simulink model "EPT"  (R2019b)
settings: Solver=FixedStepDiscrete  StartTime=0.0  StopTime=5  FixedStep=0.005  RelTol=1e-3  EnableMultiTasking=on
PreLoadFcn:
  | try, model_open; catch, disp('Error occurred while executing model pre-load callback: model_open.m'); disp('Please assure that the MATLAB working directory is set to the model directory before opening.'); end
InitFcn:
  | try, model_open; catch, end
undefined symbols (not defined in the file or in its folder): Bridge, GCM, H, ln, raptor_get_param_eval, raptor_get_safe_string, raptor_xcp_function
libraries: Raptor_lib x2810, simulink x374, hdlsllib x19
(part 6 of 45)

== system EPT/I//O/Input/ADC_CoolingSystem  ==
  raptor_analog_in1 : Raptor_lib/Input & Output/raptor_analog_in  resourceValues=INPUT2|INPUT3|INPUT4|INPUT5|INPUT6|INPUT7|INPUT8|INPUT9|INPUT10|INPUT11|INPUT12|INPUT13|INPUT14|INPUT15|INPUT16|INPUT17|INPUT18|INPUT19|INPUT20|INPUT21|INPUT22|INPUT23|INPUT24|INPUT25|INPUT26|INPUT27|INPUT28|INPUT29|INPUT30|INPUT31|INPUT32|(None)  resource=INPUT19  pullUDValues=2.15k PU  pullUD=2.15k PU  rangeValues=0 - 5 V  range=0 - 5 V  filterrateValues=[]  filterrate='RAPTOR MASK DEFAULT'  resolutionValues=[]  resolution=[]
      settings: SourceProductName=Raptor
  raptor_analog_in2 : Raptor_lib/Input & Output/raptor_analog_in  resourceValues=INPUT2|INPUT3|INPUT4|INPUT5|INPUT6|INPUT7|INPUT8|INPUT9|INPUT10|INPUT11|INPUT12|INPUT13|INPUT14|INPUT15|INPUT16|INPUT17|INPUT18|INPUT19|INPUT20|INPUT21|INPUT22|INPUT23|INPUT24|INPUT25|INPUT26|INPUT27|INPUT28|INPUT29|INPUT30|INPUT31|INPUT32|(None)  resource=INPUT3  pullUDValues=2.15k PU  pullUD=2.15k PU  rangeValues=0 - 5 V  range=0 - 5 V  filterrateValues=[]  filterrate='RAPTOR MASK DEFAULT'  resolutionValues=[]  resolution=[]
      settings: SourceProductName=Raptor
  raptor_data_def6 : Raptor_lib/Data Storage/raptor_data_def  dataName='A105_Cooling_Oil_Temp_in'  initValue=0  dataType=uint16  storage=Volatile (RAM)  calVisible=on  calType=Measurement  calDispType=Number  calEnum={'False', 'True'}  calGain=1.0  calOffset=0  calMin=-inf  calMax=inf  calFormat='-1'  calUnit=''  calHelp=''  calAccess=1  calFunction=raptor_xcp_function(gcb)  calDispHeaders=off  calColHeaders={'Col1' 'Col2' 'Col3'}  calRowHeaders={'Row1' 'Row2' 'Row3'}
      settings: SourceProductName=Raptor
  raptor_data_def9 : Raptor_lib/Data Storage/raptor_data_def  dataName='A17_Cooling_Water_Temp_in'  initValue=0  dataType=uint16  storage=Volatile (RAM)  calVisible=on  calType=Measurement  calDispType=Number  calEnum={'False', 'True'}  calGain=1.0  calOffset=0  calMin=-inf  calMax=inf  calFormat='-1'  calUnit=''  calHelp=''  calAccess=1  calFunction=raptor_xcp_function(gcb)  calDispHeaders=off  calColHeaders={'Col1' 'Col2' 'Col3'}  calRowHeaders={'Row1' 'Row2' 'Row3'}
      settings: SourceProductName=Raptor
  raptor_data_write2 : Raptor_lib/Data Storage/raptor_data_write  dataName='A17_Cooling_Water_Temp_in'  dataShape=Scalar  idxSource=Input Port  idxRow=1  idxCol=1
      settings: SourceProductName=Raptor
  raptor_data_write4 : Raptor_lib/Data Storage/raptor_data_write  dataName='A105_Cooling_Oil_Temp_in'  dataShape=Scalar  idxSource=Input Port  idxRow=1  idxCol=1
      settings: SourceProductName=Raptor
  wires:
  raptor_analog_in2/1 -> raptor_data_write2/1
  raptor_analog_in1/1 -> raptor_data_write4/1

== system EPT/I//O/Input/ADC_PlugOn ==
  raptor_analog_in : Raptor_lib/Input & Output/raptor_analog_in  resourceValues=INPUT2|INPUT3|INPUT4|INPUT5|INPUT6|INPUT7|INPUT8|INPUT9|INPUT10|INPUT11|INPUT12|INPUT13|INPUT14|INPUT15|INPUT16|INPUT17|INPUT18|INPUT19|INPUT20|INPUT21|INPUT22|INPUT23|INPUT24|INPUT25|INPUT26|INPUT27|INPUT28|INPUT29|INPUT30|INPUT31|INPUT32|(None)  resource=INPUT5  pullUDValues=681k PU  pullUD=681k PU  rangeValues=0 - 5 V  range=0 - 5 V  filterrateValues=[]  filterrate='RAPTOR MASK DEFAULT'  resolutionValues=[]  resolution=[]
      settings: SourceProductName=Raptor
  raptor_analog_in1 : Raptor_lib/Input & Output/raptor_analog_in  resourceValues=INPUT2|INPUT3|INPUT4|INPUT5|INPUT6|INPUT7|INPUT8|INPUT9|INPUT10|INPUT11|INPUT12|INPUT13|INPUT14|INPUT15|INPUT16|INPUT17|INPUT18|INPUT19|INPUT20|INPUT21|INPUT22|INPUT23|INPUT24|INPUT25|INPUT26|INPUT27|INPUT28|INPUT29|INPUT30|INPUT31|INPUT32|(None)  resource=INPUT6  pullUDValues=681k PU  pullUD=681k PU  rangeValues=0 - 5 V  range=0 - 5 V  filterrateValues=[]  filterrate='RAPTOR MASK DEFAULT'  resolutionValues=[]  resolution=[]
      settings: SourceProductName=Raptor
  raptor_measurement : Raptor_lib/Data Storage/raptor_measurement  paramName='A19_PON_SW_G2'  nameSource=Parameter  calDispType=Number  calEnum={'False', 'True'}  calGain=1.0  calOffset=0.0  calMax=inf  calMin=-inf  calFormat='-1'  calUnit=''  calHelp=''  calAccess=1  calFunction=raptor_xcp_function(gcb)  calVisible=on
      settings: SourceProductName=Raptor
  raptor_measurement1 : Raptor_lib/Data Storage/raptor_measurement  paramName='A37_PON_SW_G1'  nameSource=Parameter  calDispType=Number  calEnum={'False', 'True'}  calGain=1.0  calOffset=0.0  calMax=inf  calMin=-inf  calFormat='-1'  calUnit=''  calHelp=''  calAccess=1  calFunction=raptor_xcp_function(gcb)  calVisible=on
      settings: SourceProductName=Raptor
  wires:
  raptor_analog_in/1 -> raptor_measurement/1
  raptor_analog_in1/1 -> raptor_measurement1/1

== system EPT/I//O/Input/ADC_Reserved ==
  raptor_analog_in2 : Raptor_lib/Input & Output/raptor_analog_in  resourceValues=INPUT2|INPUT3|INPUT4|INPUT5|INPUT6|INPUT7|INPUT8|INPUT9|INPUT10|INPUT11|INPUT12|INPUT13|INPUT14|INPUT15|INPUT16|INPUT17|INPUT18|INPUT19|INPUT20|INPUT21|INPUT22|INPUT23|INPUT24|INPUT25|INPUT26|INPUT27|INPUT28|INPUT29|INPUT30|INPUT31|INPUT32|(None)  resource=INPUT8  pullUDValues=4.64k PU  pullUD=4.64k PU  rangeValues=0 - 5 V  range=0 - 5 V  filterrateValues=[]  filterrate='RAPTOR MASK DEFAULT'  resolutionValues=[]  resolution=[]
      settings: SourceProductName=Raptor
  raptor_analog_in3 : Raptor_lib/Input & Output/raptor_analog_in  resourceValues=INPUT2|INPUT3|INPUT4|INPUT5|INPUT6|INPUT7|INPUT8|INPUT9|INPUT10|INPUT11|INPUT12|INPUT13|INPUT14|INPUT15|INPUT16|INPUT17|INPUT18|INPUT19|INPUT20|INPUT21|INPUT22|INPUT23|INPUT24|INPUT25|INPUT26|INPUT27|INPUT28|INPUT29|INPUT30|INPUT31|INPUT32|(None)  resource=INPUT21  pullUDValues=2.15k PU  pullUD=2.15k PU  rangeValues=0 - 5 V  range=0 - 5 V  filterrateValues=[]  filterrate='RAPTOR MASK DEFAULT'  resolutionValues=[]  resolution=[]
      settings: SourceProductName=Raptor
  raptor_analog_in4 : Raptor_lib/Input & Output/raptor_analog_in  resourceValues=INPUT2|INPUT3|INPUT4|INPUT5|INPUT6|INPUT7|INPUT8|INPUT9|INPUT10|INPUT11|INPUT12|INPUT13|INPUT14|INPUT15|INPUT16|INPUT17|INPUT18|INPUT19|INPUT20|INPUT21|INPUT22|INPUT23|INPUT24|INPUT25|INPUT26|INPUT27|INPUT28|INPUT29|INPUT30|INPUT31|INPUT32|(None)  resource=INPUT29  pullUDValues=215k PD  pullUD=215k PD  rangeValues=0 - 5 V  range=0 - 5 V  filterrateValues=[]  filterrate='RAPTOR MASK DEFAULT'  resolutionValues=[]  resolution=[]
      settings: SourceProductName=Raptor
  raptor_measurement2 : Raptor_lib/Data Storage/raptor_measurement  paramName='A40_Position1'  nameSource=Parameter  calDispType=Number  calEnum={'False', 'True'}  calGain=1.0  calOffset=0.0  calMax=inf  calMin=-inf  calFormat='-1'  calUnit=''  calHelp=''  calAccess=1  calFunction=raptor_xcp_function(gcb)  calVisible=on
      settings: SourceProductName=Raptor
  raptor_measurement3 : Raptor_lib/Data Storage/raptor_measurement  paramName='K13_Position2'  nameSource=Parameter  calDispType=Number  calEnum={'False', 'True'}  calGain=1.0  calOffset=0.0  calMax=inf  calMin=-inf  calFormat='-1'  calUnit=''  calHelp=''  calAccess=1  calFunction=raptor_xcp_function(gcb)  calVisible=on
      settings: SourceProductName=Raptor
  raptor_measurement4 : Raptor_lib/Data Storage/raptor_measurement  paramName='K65_Mode_1'  nameSource=Parameter  calDispType=Number  calEnum={'False', 'True'}  calGain=1.0  calOffset=0.0  calMax=inf  calMin=-inf  calFormat='-1'  calUnit=''  calHelp=''  calAccess=1  calFunction=raptor_xcp_function(gcb)  calVisible=on
      settings: SourceProductName=Raptor
  wires:
  raptor_analog_in2/1 -> raptor_measurement2/1
  raptor_analog_in3/1 -> raptor_measurement3/1
  raptor_analog_in4/1 -> raptor_measurement4/1

== system EPT/I//O/Input/ADC_TemperatureBatteryPack ==
  raptor_analog_in : Raptor_lib/Input & Output/raptor_analog_in  resourceValues=INPUT2|INPUT3|INPUT4|INPUT5|INPUT6|INPUT7|INPUT8|INPUT9|INPUT10|INPUT11|INPUT12|INPUT13|INPUT14|INPUT15|INPUT16|INPUT17|INPUT18|INPUT19|INPUT20|INPUT21|INPUT22|INPUT23|INPUT24|INPUT25|INPUT26|INPUT27|INPUT28|INPUT29|INPUT30|INPUT31|INPUT32|(None)  resource=INPUT22  pullUDValues=2.15k PU  pullUD=2.15k PU  rangeValues=0 - 5 V  range=0 - 5 V  filterrateValues=[]  filterrate='RAPTOR MASK DEFAULT'  resolutionValues=[]  resolution=[]
      settings: SourceProductName=Raptor
  raptor_analog_in1 : Raptor_lib/Input & Output/raptor_analog_in  resourceValues=INPUT2|INPUT3|INPUT4|INPUT5|INPUT6|INPUT7|INPUT8|INPUT9|INPUT10|INPUT11|INPUT12|INPUT13|INPUT14|INPUT15|INPUT16|INPUT17|INPUT18|INPUT19|INPUT20|INPUT21|INPUT22|INPUT23|INPUT24|INPUT25|INPUT26|INPUT27|INPUT28|INPUT29|INPUT30|INPUT31|INPUT32|(None)  resource=INPUT25  pullUDValues=2.15k PU  pullUD=2.15k PU  rangeValues=0 - 5 V  range=0 - 5 V  filterrateValues=[]  filterrate='RAPTOR MASK DEFAULT'  resolutionValues=[]  resolution=[]
      settings: SourceProductName=Raptor
  raptor_analog_in2 : Raptor_lib/Input & Output/raptor_analog_in  resourceValues=INPUT2|INPUT3|INPUT4|INPUT5|INPUT6|INPUT7|INPUT8|INPUT9|INPUT10|INPUT11|INPUT12|INPUT13|INPUT14|INPUT15|INPUT16|INPUT17|INPUT18|INPUT19|INPUT20|INPUT21|INPUT22|INPUT23|INPUT24|INPUT25|INPUT26|INPUT27|INPUT28|INPUT29|INPUT30|INPUT31|INPUT32|(None)  resource=INPUT27  pullUDValues=2.15k PU  pullUD=2.15k PU  rangeValues=0 - 5 V  range=0 - 5 V  filterrateValues=[]  filterrate='RAPTOR MASK DEFAULT'  resolutionValues=[]  resolution=[]
      settings: SourceProductName=Raptor
  raptor_analog_in3 : Raptor_lib/Input & Output/raptor_analog_in  resourceValues=INPUT2|INPUT3|INPUT4|INPUT5|INPUT6|INPUT7|INPUT8|INPUT9|INPUT10|INPUT11|INPUT12|INPUT13|INPUT14|INPUT15|INPUT16|INPUT17|INPUT18|INPUT19|INPUT20|INPUT21|INPUT22|INPUT23|INPUT24|INPUT25|INPUT26|INPUT27|INPUT28|INPUT29|INPUT30|INPUT31|INPUT32|(None)  resource=INPUT28  pullUDValues=2.15k PU  pullUD=2.15k PU  rangeValues=0 - 5 V  range=0 - 5 V  filterrateValues=[]  filterrate='RAPTOR MASK DEFAULT'  resolutionValues=[]  resolution=[]
      settings: SourceProductName=Raptor
  raptor_data_def : Raptor_lib/Data Storage/raptor_data_def  dataName='TBP_2'  initValue=0  dataType=uint16  storage=Volatile (RAM)  calVisible=on  calType=Measurement  calDispType=Number  calEnum={'False', 'True'}  calGain=1.0  calOffset=0  calMin=-inf  calMax=inf  calFormat='-1'  calUnit=''  calHelp=''  calAccess=1  calFunction=raptor_xcp_function(gcb)  calDispHeaders=off  calColHeaders={'Col1' 'Col2' 'Col3'}  calRowHeaders={'Row1' 'Row2' 'Row3'}
      settings: SourceProductName=Raptor
  raptor_data_def1 : Raptor_lib/Data Storage/raptor_data_def  dataName='TBP_1'  initValue=0  dataType=uint16  storage=Volatile (RAM)  calVisible=on  calType=Measurement  calDispType=Number  calEnum={'False', 'True'}  calGain=1.0  calOffset=0  calMin=-inf  calMax=inf  calFormat='-1'  calUnit=''  calHelp=''  calAccess=1  calFunction=raptor_xcp_function(gcb)  calDispHeaders=off  calColHeaders={'Col1' 'Col2' 'Col3'}  calRowHeaders={'Row1' 'Row2' 'Row3'}
      settings: SourceProductName=Raptor
  raptor_data_def2 : Raptor_lib/Data Storage/raptor_data_def  dataName='TBP_3'  initValue=0  dataType=uint16  storage=Volatile (RAM)  calVisible=on  calType=Measurement  calDispType=Number  calEnum={'False', 'True'}  calGain=1.0  calOffset=0  calMin=-inf  calMax=inf  calFormat='-1'  calUnit=''  calHelp=''  calAccess=1  calFunction=raptor_xcp_function(gcb)  calDispHeaders=off  calColHeaders={'Col1' 'Col2' 'Col3'}  calRowHeaders={'Row1' 'Row2' 'Row3'}
      settings: SourceProductName=Raptor
  raptor_data_def3 : Raptor_lib/Data Storage/raptor_data_def  dataName='TBP_4'  initValue=0  dataType=uint16  storage=Volatile (RAM)  calVisible=on  calType=Measurement  calDispType=Number  calEnum={'False', 'True'}  calGain=1.0  calOffset=0  calMin=-inf  calMax=inf  calFormat='-1'  calUnit=''  calHelp=''  calAccess=1  calFunction=raptor_xcp_function(gcb)  calDispHeaders=off  calColHeaders={'Col1' 'Col2' 'Col3'}  calRowHeaders={'Row1' 'Row2' 'Row3'}
      settings: SourceProductName=Raptor
  raptor_data_write1 : Raptor_lib/Data Storage/raptor_data_write  dataName='TBP_1'  dataShape=Scalar  idxSource=Input Port  idxRow=1  idxCol=1
      settings: SourceProductName=Raptor
  raptor_data_write2 : Raptor_lib/Data Storage/raptor_data_write  dataName='TBP_2'  dataShape=Scalar  idxSource=Input Port  idxRow=1  idxCol=1
      settings: SourceProductName=Raptor
  raptor_data_write3 : Raptor_lib/Data Storage/raptor_data_write  dataName='TBP_3'  dataShape=Scalar  idxSource=Input Port  idxRow=1  idxCol=1
      settings: SourceProductName=Raptor
  raptor_data_write4 : Raptor_lib/Data Storage/raptor_data_write  dataName='TBP_4'  dataShape=Scalar  idxSource=Input Port  idxRow=1  idxCol=1
      settings: SourceProductName=Raptor
  raptor_measurement : Raptor_lib/Data Storage/raptor_measurement  paramName='K30_TBP_1'  nameSource=Parameter  calDispType=Number  calEnum={'False', 'True'}  calGain=1.0  calOffset=0.0  calMax=inf  calMin=-inf  calFormat='-1'  calUnit=''  calHelp=''  calAccess=1  calFunction=raptor_xcp_function(gcb)  calVisible=on
      settings: SourceProductName=Raptor
  raptor_measurement1 : Raptor_lib/Data Storage/raptor_measurement  paramName='K42_TBP_2'  nameSource=Parameter  calDispType=Number  calEnum={'False', 'True'}  calGain=1.0  calOffset=0.0  calMax=inf  calMin=-inf  calFormat='-1'  calUnit=''  calHelp=''  calAccess=1  calFunction=raptor_xcp_function(gcb)  calVisible=on
      settings: SourceProductName=Raptor
  raptor_measurement2 : Raptor_lib/Data Storage/raptor_measurement  paramName='K51_TBP_3'  nameSource=Parameter  calDispType=Number  calEnum={'False', 'True'}  calGain=1.0  calOffset=0.0  calMax=inf  calMin=-inf  calFormat='-1'  calUnit=''  calHelp=''  calAccess=1  calFunction=raptor_xcp_function(gcb)  calVisible=on
      settings: SourceProductName=Raptor
  raptor_measurement3 : Raptor_lib/Data Storage/raptor_measurement  paramName='K58_TBP_4'  nameSource=Parameter  calDispType=Number  calEnum={'False', 'True'}  calGain=1.0  calOffset=0.0  calMax=inf  calMin=-inf  calFormat='-1'  calUnit=''  calHelp=''  calAccess=1  calFunction=raptor_xcp_function(gcb)  calVisible=on
      settings: SourceProductName=Raptor
  wires:
  raptor_analog_in/1 -> raptor_data_write1/1, raptor_measurement/1
  raptor_analog_in3/1 -> raptor_data_write4/1, raptor_measurement3/1
  raptor_analog_in2/1 -> raptor_measurement2/1, raptor_data_write3/1
  raptor_analog_in1/1 -> raptor_measurement1/1, raptor_data_write2/1

== system EPT/I//O/Input/Curtis_Reserved  ==
  raptor_analog_in : Raptor_lib/Input & Output/raptor_analog_in  resourceValues=INPUT2|INPUT3|INPUT4|INPUT5|INPUT6|INPUT7|INPUT8|INPUT9|INPUT10|INPUT11|INPUT12|INPUT13|INPUT14|INPUT15|INPUT16|INPUT17|INPUT18|INPUT19|INPUT20|INPUT21|INPUT22|INPUT23|INPUT24|INPUT25|INPUT26|INPUT27|INPUT28|INPUT29|INPUT30|INPUT31|INPUT32|(None)  resource=INPUT11  pullUDValues=681k PU  pullUD=681k PU  rangeValues=0 - 5 V  range=0 - 5 V  filterrateValues=[]  filterrate='RAPTOR MASK DEFAULT'  resolutionValues=[]  resolution=[]
      settings: SourceProductName=Raptor
  raptor_freq_in : Raptor_lib/Input & Output/raptor_freq_in  resourceValues=INPUT41|INPUT42|INPUT43|INPUT44|INPUT45|(None)  resource=INPUT42  hasDuty=on  pullUDValues=[]  pullUD=[]  interfaceValues=[]  interface=[]  hasEdgeCount='RAPTOR MASK DEFAULT'  filterValues=[]  filter=[]
      settings: SourceProductName=Raptor
  raptor_freq_in1 : Raptor_lib/Input & Output/raptor_freq_in  resourceValues=INPUT41|INPUT42|INPUT43|INPUT44|INPUT45|(None)  resource=INPUT45  hasDuty=on  pullUDValues=[]  pullUD=[]  interfaceValues=[]  interface=[]  hasEdgeCount='RAPTOR MASK DEFAULT'  filterValues=[]  filter=[]
      settings: SourceProductName=Raptor
  raptor_measurement : Raptor_lib/Data Storage/raptor_measurement  paramName='A55_MCU_Mode'  nameSource=Parameter  calDispType=Number  calEnum={'False', 'True'}  calGain=1.0  calOffset=0.0  calMax=inf  calMin=-inf  calFormat='-1'  calUnit=''  calHelp=''  calAccess=1  calFunction=raptor_xcp_function(gcb)  calVisible=on
      settings: SourceProductName=Raptor
  raptor_measurement1 : Raptor_lib/Data Storage/raptor_measurement  paramName='K18_Freq_MrpmA'  nameSource=Parameter  calDispType=Number  calEnum={'False', 'True'}  calGain=1.0  calOffset=0.0  calMax=inf  calMin=-inf  calFormat='-1'  calUnit=''  calHelp=''  calAccess=1  calFunction=raptor_xcp_function(gcb)  calVisible=on
      settings: SourceProductName=Raptor
  raptor_measurement2 : Raptor_lib/Data Storage/raptor_measurement  paramName='K52_Freq_MrpmB'  nameSource=Parameter  calDispType=Number  calEnum={'False', 'True'}  calGain=1.0  calOffset=0.0  calMax=inf  calMin=-inf  calFormat='-1'  calUnit=''  calHelp=''  calAccess=1  calFunction=raptor_xcp_function(gcb)  calVisible=on
      settings: SourceProductName=Raptor
  raptor_measurement3 : Raptor_lib/Data Storage/raptor_measurement  paramName='K18_Duty_MrpmA'  nameSource=Parameter  calDispType=Number  calEnum={'False', 'True'}  calGain=1.0  calOffset=0.0  calMax=inf  calMin=-inf  calFormat='-1'  calUnit=''  calHelp=''  calAccess=1  calFunction=raptor_xcp_function(gcb)  calVisible=on
      settings: SourceProductName=Raptor
  raptor_measurement5 : Raptor_lib/Data Storage/raptor_measurement  paramName='K52_Duty_MrpmB'  nameSource=Parameter  calDispType=Number  calEnum={'False', 'True'}  calGain=1.0  calOffset=0.0  calMax=inf  calMin=-inf  calFormat='-1'  calUnit=''  calHelp=''  calAccess=1  calFunction=raptor_xcp_function(gcb)  calVisible=on
      settings: SourceProductName=Raptor
  wires:
  raptor_analog_in/1 -> raptor_measurement/1
  raptor_freq_in/1 -> raptor_measurement1/1
  raptor_freq_in1/1 -> raptor_measurement2/1
  raptor_freq_in/2 -> raptor_measurement3/1
  raptor_freq_in1/2 -> raptor_measurement5/1

== system EPT/I//O/Output/BatteryPack_RelayControl  ==
  raptor_data_def16 : Raptor_lib/Data Storage/raptor_data_def  dataName='Flag_HV_Negative_Relay_On'  initValue=0  dataType=boolean  storage=Volatile (RAM)  calVisible=on  calType=Measurement  calDispType=Number  calEnum={'False', 'True'}  calGain=1.0  calOffset=0  calMin=-inf  calMax=inf  calFormat='-1'  calUnit=''  calHelp=''  calAccess=1  calFunction=raptor_xcp_function(gcb)  calDispHeaders=off  calColHeaders={'Col1' 'Col2' 'Col3'}  calRowHeaders={'Row1' 'Row2' 'Row3'}
      settings: SourceProductName=Raptor
  raptor_data_def17 : Raptor_lib/Data Storage/raptor_data_def  dataName='Flag_HV_Drive_Relay_On'  initValue=0  dataType=boolean  storage=Volatile (RAM)  calVisible=on  calType=Measurement  calDispType=Number  calEnum={'False', 'True'}  calGain=1.0  calOffset=0  calMin=-inf  calMax=inf  calFormat='-1'  calUnit=''  calHelp=''  calAccess=1  calFunction=raptor_xcp_function(gcb)  calDispHeaders=off  calColHeaders={'Col1' 'Col2' 'Col3'}  calRowHeaders={'Row1' 'Row2' 'Row3'}
      settings: SourceProductName=Raptor
  raptor_data_def18 : Raptor_lib/Data Storage/raptor_data_def  dataName='Flag_PreCharge_Relay_On'  initValue=0  dataType=boolean  storage=Volatile (RAM)  calVisible=on  calType=Measurement  calDispType=Number  calEnum={'False', 'True'}  calGain=1.0  calOffset=0  calMin=-inf  calMax=inf  calFormat='-1'  calUnit=''  calHelp=''  calAccess=1  calFunction=raptor_xcp_function(gcb)  calDispHeaders=off  calColHeaders={'Col1' 'Col2' 'Col3'}  calRowHeaders={'Row1' 'Row2' 'Row3'}
      settings: SourceProductName=Raptor
  raptor_data_def19 : Raptor_lib/Data Storage/raptor_data_def  dataName='Flag_Charger_Relay_On'  initValue=0  dataType=boolean  storage=Volatile (RAM)  calVisible=on  calType=Measurement  calDispType=Number  calEnum={'False', 'True'}  calGain=1.0  calOffset=0  calMin=-inf  calMax=inf  calFormat='-1'  calUnit=''  calHelp=''  calAccess=1  calFunction=raptor_xcp_function(gcb)  calDispHeaders=off  calColHeaders={'Col1' 'Col2' 'Col3'}  calRowHeaders={'Row1' 'Row2' 'Row3'}
      settings: SourceProductName=Raptor
  raptor_data_read1 : Raptor_lib/Data Storage/raptor_data_read  dataName='Flag_HV_Drive_Relay_On'  dataShape=Scalar  idxSource=Input  idxRow=1  idxCol=1
      settings: SourceProductName=Raptor
  raptor_data_read2 : Raptor_lib/Data Storage/raptor_data_read  dataName='Flag_PreCharge_Relay_On'  dataShape=Scalar  idxSource=Input  idxRow=1  idxCol=1
      settings: SourceProductName=Raptor
  raptor_data_read3 : Raptor_lib/Data Storage/raptor_data_read  dataName='Flag_Charger_Relay_On'  dataShape=Scalar  idxSource=Input  idxRow=1  idxCol=1
      settings: SourceProductName=Raptor
  raptor_data_read4 : Raptor_lib/Data Storage/raptor_data_read  dataName='Flag_HV_Negative_Relay_On'  dataShape=Scalar  idxSource=Input  idxRow=1  idxCol=1
      settings: SourceProductName=Raptor
  raptor_digital_out : Raptor_lib/Input & Output/raptor_digital_out  resourceValues=OUTPUT1|OUTPUT2|OUTPUT3|OUTPUT4|OUTPUT5|OUTPUT6|OUTPUT7|OUTPUT8|OUTPUT9|OUTPUT10|OUTPUT11|OUTPUT12|OUTPUT21|OUTPUT22|OUTPUT23|OUTPUT24|OUTPUT25|OUTPUT26|OUTPUT27|OUTPUT28|OUTPUT29|OUTPUT30|OUTPUT31|OUTPUT32|OUTPUT33|OUTPUT34|OUTPUT35|OUTPUT36|OUTPUT37|OUTPUT38|OUTPUT39|OUTPUT40|OUTPUT41|OUTPUT42|OUTPUT43|OUTPUT44|OUTPUT45|OUTPUT46|OUTPUT47|OUTPUT48|OUTPUT49|POWER_HOLD|(None)  resource=OUTPUT9  driverTypeValues=Low Side  driverType=Low Side
      settings: SourceProductName=Raptor
  raptor_digital_out1 : Raptor_lib/Input & Output/raptor_digital_out  resourceValues=OUTPUT1|OUTPUT2|OUTPUT3|OUTPUT4|OUTPUT5|OUTPUT6|OUTPUT7|OUTPUT8|OUTPUT9|OUTPUT10|OUTPUT11|OUTPUT12|OUTPUT21|OUTPUT22|OUTPUT23|OUTPUT24|OUTPUT25|OUTPUT26|OUTPUT27|OUTPUT28|OUTPUT29|OUTPUT30|OUTPUT31|OUTPUT32|OUTPUT33|OUTPUT34|OUTPUT35|OUTPUT36|OUTPUT37|OUTPUT38|OUTPUT39|OUTPUT40|OUTPUT41|OUTPUT42|OUTPUT43|OUTPUT44|OUTPUT45|OUTPUT46|OUTPUT47|OUTPUT48|OUTPUT49|POWER_HOLD|(None)  resource=OUTPUT12  driverTypeValues=Low Side  driverType=Low Side
      settings: SourceProductName=Raptor
  raptor_digital_out2 : Raptor_lib/Input & Output/raptor_digital_out  resourceValues=OUTPUT1|OUTPUT2|OUTPUT3|OUTPUT4|OUTPUT5|OUTPUT6|OUTPUT7|OUTPUT8|OUTPUT9|OUTPUT10|OUTPUT11|OUTPUT12|OUTPUT21|OUTPUT22|OUTPUT23|OUTPUT24|OUTPUT25|OUTPUT26|OUTPUT27|OUTPUT28|OUTPUT29|OUTPUT30|OUTPUT31|OUTPUT32|OUTPUT33|OUTPUT34|OUTPUT35|OUTPUT36|OUTPUT37|OUTPUT38|OUTPUT39|OUTPUT40|OUTPUT41|OUTPUT42|OUTPUT43|OUTPUT44|OUTPUT45|OUTPUT46|OUTPUT47|OUTPUT48|OUTPUT49|POWER_HOLD|(None)  resource=OUTPUT10  driverTypeValues=Low Side  driverType=Low Side
      settings: SourceProductName=Raptor
  raptor_digital_out3 : Raptor_lib/Input & Output/raptor_digital_out  resourceValues=OUTPUT1|OUTPUT2|OUTPUT3|OUTPUT4|OUTPUT5|OUTPUT6|OUTPUT7|OUTPUT8|OUTPUT9|OUTPUT10|OUTPUT11|OUTPUT12|OUTPUT21|OUTPUT22|OUTPUT23|OUTPUT24|OUTPUT25|OUTPUT26|OUTPUT27|OUTPUT28|OUTPUT29|OUTPUT30|OUTPUT31|OUTPUT32|OUTPUT33|OUTPUT34|OUTPUT35|OUTPUT36|OUTPUT37|OUTPUT38|OUTPUT39|OUTPUT40|OUTPUT41|OUTPUT42|OUTPUT43|OUTPUT44|OUTPUT45|OUTPUT46|OUTPUT47|OUTPUT48|OUTPUT49|POWER_HOLD|(None)  resource=OUTPUT21  driverTypeValues=Low Side  driverType=Low Side
      settings: SourceProductName=Raptor
  raptor_override1 : Raptor_lib/Data Storage/raptor_override  paramName='Cal_Relay_Drive'  nameSource=Parameter  measurement=None  calDispType=Number  calEnum={'False', 'True'}  calGain=1.0  calOffset=0.0  calMax=inf  calMin=-inf  calFormat='-1'  calUnit=''  calHelp=''  calAccess=1  calFunction=[raptor_xcp_function(gcb) '|' raptor_get_param_eval(gcb, 'paramName') '_Override']
      settings: SourceProductName=Raptor
  raptor_override2 : Raptor_lib/Data Storage/raptor_override  paramName='Cal_Relay_HV_Negative'  nameSource=Parameter  measurement=None  calDispType=Number  calEnum={'False', 'True'}  calGain=1.0  calOffset=0.0  calMax=inf  calMin=-inf  calFormat='-1'  calUnit=''  calHelp=''  calAccess=1  calFunction=[raptor_xcp_function(gcb) '|' raptor_get_param_eval(gcb, 'paramName') '_Override']
      settings: SourceProductName=Raptor
  raptor_override3 : Raptor_lib/Data Storage/raptor_override  paramName='Cal_Relay_PreChg'  nameSource=Parameter  measurement=None  calDispType=Number  calEnum={'False', 'True'}  calGain=1.0  calOffset=0.0  calMax=inf  calMin=-inf  calFormat='-1'  calUnit=''  calHelp=''  calAccess=1  calFunction=[raptor_xcp_function(gcb) '|' raptor_get_param_eval(gcb, 'paramName') '_Override']
      settings: SourceProductName=Raptor
  raptor_override4 : Raptor_lib/Data Storage/raptor_override  paramName='Cal_Relay_CHG'  nameSource=Parameter  measurement=None  calDispType=Number  calEnum={'False', 'True'}  calGain=1.0  calOffset=0.0  calMax=inf  calMin=-inf  calFormat='-1'  calUnit=''  calHelp=''  calAccess=1  calFunction=[raptor_xcp_function(gcb) '|' raptor_get_param_eval(gcb, 'paramName') '_Override']
      settings: SourceProductName=Raptor
  wires:
  raptor_data_read4/1 -> raptor_override2/1
  raptor_data_read2/1 -> raptor_override3/1
  raptor_override2/1 -> raptor_digital_out/1
  raptor_data_read1/1 -> raptor_override1/1
  raptor_override3/1 -> raptor_digital_out2/1
  raptor_override4/1 -> raptor_digital_out3/1
  raptor_data_read3/1 -> raptor_override4/1
  raptor_override1/1 -> raptor_digital_out1/1

== system EPT/I//O/Output/ChargerPlugInterface ==
  note: CHG Enable
  note: EOC Enable
  raptor_data_def13 : Raptor_lib/Data Storage/raptor_data_def  dataName='A24_EOC_Enable'  initValue=0  dataType=boolean  storage=Volatile (RAM)  calVisible=on  calType=Measurement  calDispType=Number  calEnum={'False', 'True'}  calGain=1.0  calOffset=0  calMin=-inf  calMax=inf  calFormat='-1'  calUnit=''  calHelp=''  calAccess=1  calFunction=raptor_xcp_function(gcb)  calDispHeaders=off  calColHeaders={'Col1' 'Col2' 'Col3'}  calRowHeaders={'Row1' 'Row2' 'Row3'}
      settings: SourceProductName=Raptor
  raptor_data_def14 : Raptor_lib/Data Storage/raptor_data_def  dataName='A10_CHG_Enable'  initValue=0  dataType=boolean  storage=Volatile (RAM)  calVisible=on  calType=Measurement  calDispType=Number  calEnum={'False', 'True'}  calGain=1.0  calOffset=0  calMin=-inf  calMax=inf  calFormat='-1'  calUnit=''  calHelp=''  calAccess=1  calFunction=raptor_xcp_function(gcb)  calDispHeaders=off  calColHeaders={'Col1' 'Col2' 'Col3'}  calRowHeaders={'Row1' 'Row2' 'Row3'}
      settings: SourceProductName=Raptor
  raptor_data_read1 : Raptor_lib/Data Storage/raptor_data_read  dataName='A24_EOC_Enable'  dataShape=Scalar  idxSource=Input  idxRow=1  idxCol=1
      settings: SourceProductName=Raptor
  raptor_data_read4 : Raptor_lib/Data Storage/raptor_data_read  dataName='A10_CHG_Enable'  dataShape=Scalar  idxSource=Input  idxRow=1  idxCol=1
      settings: SourceProductName=Raptor
  raptor_digital_out3 : Raptor_lib/Input & Output/raptor_digital_out  resourceValues=OUTPUT1|OUTPUT2|OUTPUT3|OUTPUT4|OUTPUT5|OUTPUT6|OUTPUT7|OUTPUT8|OUTPUT9|OUTPUT10|OUTPUT11|OUTPUT12|OUTPUT21|OUTPUT22|OUTPUT23|OUTPUT24|OUTPUT25|OUTPUT26|OUTPUT27|OUTPUT28|OUTPUT29|OUTPUT30|OUTPUT31|OUTPUT32|OUTPUT33|OUTPUT34|OUTPUT35|OUTPUT36|OUTPUT37|OUTPUT38|OUTPUT39|OUTPUT40|OUTPUT41|OUTPUT42|OUTPUT43|OUTPUT44|OUTPUT45|OUTPUT46|OUTPUT47|OUTPUT48|OUTPUT49|POWER_HOLD|(None)  resource=OUTPUT1  driverTypeValues=Low Side  driverType=Low Side
      settings: SourceProductName=Raptor
  raptor_digital_out4 : Raptor_lib/Input & Output/raptor_digital_out  resourceValues=OUTPUT1|OUTPUT2|OUTPUT3|OUTPUT4|OUTPUT5|OUTPUT6|OUTPUT7|OUTPUT8|OUTPUT9|OUTPUT10|OUTPUT11|OUTPUT12|OUTPUT21|OUTPUT22|OUTPUT23|OUTPUT24|OUTPUT25|OUTPUT26|OUTPUT27|OUTPUT28|OUTPUT29|OUTPUT30|OUTPUT31|OUTPUT32|OUTPUT33|OUTPUT34|OUTPUT35|OUTPUT36|OUTPUT37|OUTPUT38|OUTPUT39|OUTPUT40|OUTPUT41|OUTPUT42|OUTPUT43|OUTPUT44|OUTPUT45|OUTPUT46|OUTPUT47|OUTPUT48|OUTPUT49|POWER_HOLD|(None)  resource=OUTPUT3  driverTypeValues=Low Side  driverType=Low Side
      settings: SourceProductName=Raptor
  raptor_override : Raptor_lib/Data Storage/raptor_override  paramName='Cal_CHG_Enable'  nameSource=Parameter  measurement=None  calDispType=Number  calEnum={'False', 'True'}  calGain=1.0  calOffset=0.0  calMax=inf  calMin=-inf  calFormat='-1'  calUnit=''  calHelp=''  calAccess=1  calFunction=[raptor_xcp_function(gcb) '|' raptor_get_param_eval(gcb, 'paramName') '_Override']
      settings: SourceProductName=Raptor
  raptor_override1 : Raptor_lib/Data Storage/raptor_override  paramName='Cal_EOC_Enable'  nameSource=Parameter  measurement=None  calDispType=Number  calEnum={'False', 'True'}  calGain=1.0  calOffset=0.0  calMax=inf  calMin=-inf  calFormat='-1'  calUnit=''  calHelp=''  calAccess=1  calFunction=[raptor_xcp_function(gcb) '|' raptor_get_param_eval(gcb, 'paramName') '_Override']
      settings: SourceProductName=Raptor
  wires:
  raptor_data_read4/1 -> raptor_override/1
  raptor_data_read1/1 -> raptor_override1/1
  raptor_override/1 -> raptor_digital_out3/1
  raptor_override1/1 -> raptor_digital_out4/1

== system EPT/I//O/Output/Cooling System ==
  note: Motor Cooling
  note: OIL COOLER FAN
  note: WATER COOLER FAN
  note: MOTOR COOLER PW
  note: PACK COOLER PW
  note: Pack Cooling
  note: OIL COOLER FAN
  note: OIL PUMP
  note: WATER PUMP
  Data Type Conversion{,1..5} (6 alike) : DataTypeConversion
  Gain1 : Gain  Gain=100  OutDataTypeStr=uint32
  Gain2 : Gain  Gain=100  OutDataTypeStr=uint16
  Gain3 : Gain  Gain=100  OutDataTypeStr=uint32
  Gain4 : Gain  Gain=100  OutDataTypeStr=uint16
  Gain5 : Gain  Gain=100  OutDataTypeStr=uint32
  Gain6 : Gain  Gain=100  OutDataTypeStr=uint16
  raptor_adjustment1 : Raptor_lib/Data Storage/raptor_adjustment  paramName='K88_LSD_PWM_Freq'  nameSource=Parameter  initValue=1000  dataType=uint32  storage=Calibration  calDispType=Number  calEnum={'False', 'True'}  calGain=1.0  calOffset=0.0  calMax=inf  calMin=-inf  calFormat='-1'  calUnit=''  calHelp=''  calAccess=1  calFunction=raptor_xcp_function(gcb)  calDispHeaders=off  calColHeaders={'Col1' 'Col2' 'Col3'}  calRowHeaders={'Row1' 'Row2' 'Row3'}
      settings: SourceProductName=Raptor
  raptor_adjustment2 : Raptor_lib/Data Storage/raptor_adjustment  paramName='K88_LSD_PWM_EN'  nameSource=Parameter  initValue=1  dataType=boolean  storage=Calibration  calDispType=Number  calEnum={'False', 'True'}  calGain=1.0  calOffset=0.0  calMax=inf  calMin=-inf  calFormat='-1'  calUnit=''  calHelp=''  calAccess=1  calFunction=raptor_xcp_function(gcb)  calDispHeaders=off  calColHeaders={'Col1' 'Col2' 'Col3'}  calRowHeaders={'Row1' 'Row2' 'Row3'}
      settings: SourceProductName=Raptor
  raptor_adjustment3 : Raptor_lib/Data Storage/raptor_adjustment  paramName='A93_LSD_PWM_EN'  nameSource=Parameter  initValue=1  dataType=boolean  storage=Calibration  calDispType=Number  calEnum={'False', 'True'}  calGain=1.0  calOffset=0.0  calMax=inf  calMin=-inf  calFormat='-1'  calUnit=''  calHelp=''  calAccess=1  calFunction=raptor_xcp_function(gcb)  calDispHeaders=off  calColHeaders={'Col1' 'Col2' 'Col3'}  calRowHeaders={'Row1' 'Row2' 'Row3'}
      settings: SourceProductName=Raptor
  raptor_adjustment6 : Raptor_lib/Data Storage/raptor_adjustment  paramName='A23_LSD_PWM_Freq'  nameSource=Parameter  initValue=1000  dataType=uint32  storage=Calibration  calDispType=Number  calEnum={'False', 'True'}  calGain=1.0  calOffset=0.0  calMax=inf  calMin=-inf  calFormat='-1'  calUnit=''  calHelp=''  calAccess=1  calFunction=raptor_xcp_function(gcb)  calDispHeaders=off  calColHeaders={'Col1' 'Col2' 'Col3'}  calRowHeaders={'Row1' 'Row2' 'Row3'}
      settings: SourceProductName=Raptor
  raptor_adjustment7 : Raptor_lib/Data Storage/raptor_adjustment  paramName='A23_LSD_PWM_EN'  nameSource=Parameter  initValue=1  dataType=boolean  storage=Calibration  calDispType=Number  calEnum={'False', 'True'}  calGain=1.0  calOffset=0.0  calMax=inf  calMin=-inf  calFormat='-1'  calUnit=''  calHelp=''  calAccess=1  calFunction=raptor_xcp_function(gcb)  calDispHeaders=off  calColHeaders={'Col1' 'Col2' 'Col3'}  calRowHeaders={'Row1' 'Row2' 'Row3'}
      settings: SourceProductName=Raptor
  raptor_adjustment8 : Raptor_lib/Data Storage/raptor_adjustment  paramName='A93_LSD_PWM_Freq'  nameSource=Parameter  initValue=1000  dataType=uint32  storage=Calibration  calDispType=Number  calEnum={'False', 'True'}  calGain=1.0  calOffset=0.0  calMax=inf  calMin=-inf  calFormat='-1'  calUnit=''  calHelp=''  calAccess=1  calFunction=raptor_xcp_function(gcb)  calDispHeaders=off  calColHeaders={'Col1' 'Col2' 'Col3'}  calRowHeaders={'Row1' 'Row2' 'Row3'}
      settings: SourceProductName=Raptor
  raptor_data_def : Raptor_lib/Data Storage/raptor_data_def  dataName='A93_LSD_PWM_Duty'  initValue=0  dataType=double  storage=Volatile (RAM)  calVisible=on  calType=Measurement  calDispType=Number  calEnum={'False', 'True'}  calGain=1.0  calOffset=0  calMin=-inf  calMax=inf  calFormat='-1'  calUnit=''  calHelp=''  calAccess=1  calFunction=raptor_xcp_function(gcb)  calDispHeaders=off  calColHeaders={'Col1' 'Col2' 'Col3'}  calRowHeaders={'Row1' 'Row2' 'Row3'}
      settings: SourceProductName=Raptor
  raptor_data_def1 : Raptor_lib/Data Storage/raptor_data_def  dataName='K19_LSD_Relay_EAU2'  initValue=0  dataType=boolean  storage=Volatile (RAM)  calVisible=on  calType=Measurement  calDispType=Number  calEnum={'False', 'True'}  calGain=1.0  calOffset=0  calMin=-inf  calMax=inf  calFormat='-1'  calUnit=''  calHelp=''  calAccess=1  calFunction=raptor_xcp_function(gcb)  calDispHeaders=off  calColHeaders={'Col1' 'Col2' 'Col3'}  calRowHeaders={'Row1' 'Row2' 'Row3'}
      settings: SourceProductName=Raptor
  raptor_data_def2 : Raptor_lib/Data Storage/raptor_data_def  dataName='A23_LSD_PWM_Duty'  initValue=0  dataType=double  storage=Calibration  calVisible=on  calType=Measurement  calDispType=Number  calEnum={'False', 'True'}  calGain=1.0  calOffset=0  calMin=-inf  calMax=inf  calFormat='-1'  calUnit=''  calHelp=''  calAccess=1  calFunction=raptor_xcp_function(gcb)  calDispHeaders=off  calColHeaders={'Col1' 'Col2' 'Col3'}  calRowHeaders={'Row1' 'Row2' 'Row3'}
      settings: SourceProductName=Raptor
  raptor_data_def3 : Raptor_lib/Data Storage/raptor_data_def  dataName='A46_LSD_Relay_OC'  initValue=0  dataType=boolean  storage=Volatile (RAM)  calVisible=on  calType=Measurement  calDispType=Number  calEnum={'False', 'True'}  calGain=1.0  calOffset=0  calMin=-inf  calMax=inf  calFormat='-1'  calUnit=''  calHelp=''  calAccess=1  calFunction=raptor_xcp_function(gcb)  calDispHeaders=off  calColHeaders={'Col1' 'Col2' 'Col3'}  calRowHeaders={'Row1' 'Row2' 'Row3'}
      settings: SourceProductName=Raptor
  raptor_data_def4 : Raptor_lib/Data Storage/raptor_data_def  dataName='K55_LSD_Relay_WC'  initValue=0  dataType=boolean  storage=Volatile (RAM)  calVisible=on  calType=Measurement  calDispType=Number  calEnum={'False', 'True'}  calGain=1.0  calOffset=0  calMin=-inf  calMax=inf  calFormat='-1'  calUnit=''  calHelp=''  calAccess=1  calFunction=raptor_xcp_function(gcb)  calDispHeaders=off  calColHeaders={'Col1' 'Col2' 'Col3'}  calRowHeaders={'Row1' 'Row2' 'Row3'}
      settings: SourceProductName=Raptor
  raptor_data_def5 : Raptor_lib/Data Storage/raptor_data_def  dataName='K88_LSD_PWM_Duty'  initValue=0  dataType=double  storage=Calibration  calVisible=on  calType=Measurement  calDispType=Number  calEnum={'False', 'True'}  calGain=1.0  calOffset=0  calMin=-inf  calMax=inf  calFormat='-1'  calUnit=''  calHelp=''  calAccess=1  calFunction=raptor_xcp_function(gcb)  calDispHeaders=off  calColHeaders={'Col1' 'Col2' 'Col3'}  calRowHeaders={'Row1' 'Row2' 'Row3'}
      settings: SourceProductName=Raptor
  raptor_data_def7 : Raptor_lib/Data Storage/raptor_data_def  dataName='K37_LSD_Relay_EAU1'  initValue=0  dataType=boolean  storage=Volatile (RAM)  calVisible=on  calType=Measurement  calDispType=Number  calEnum={'False', 'True'}  calGain=1.0  calOffset=0  calMin=-inf  calMax=inf  calFormat='-1'  calUnit=''  calHelp=''  calAccess=1  calFunction=raptor_xcp_function(gcb)  calDispHeaders=off  calColHeaders={'Col1' 'Col2' 'Col3'}  calRowHeaders={'Row1' 'Row2' 'Row3'}
      settings: SourceProductName=Raptor
  raptor_data_read : Raptor_lib/Data Storage/raptor_data_read  dataName='A93_LSD_PWM_Duty'  dataShape=Scalar  idxSource=Input  idxRow=1  idxCol=1
      settings: SourceProductName=Raptor
  raptor_data_read1 : Raptor_lib/Data Storage/raptor_data_read  dataName='A23_LSD_PWM_Duty'  dataShape=Scalar  idxSource=Input  idxRow=1  idxCol=1
      settings: SourceProductName=Raptor
  raptor_data_read2 : Raptor_lib/Data Storage/raptor_data_read  dataName='A46_LSD_Relay_OC'  dataShape=Scalar  idxSource=Input  idxRow=1  idxCol=1
      settings: SourceProductName=Raptor
  raptor_data_read3 : Raptor_lib/Data Storage/raptor_data_read  dataName='K55_LSD_Relay_WC'  dataShape=Scalar  idxSource=Input  idxRow=1  idxCol=1
      settings: SourceProductName=Raptor
  raptor_data_read4 : Raptor_lib/Data Storage/raptor_data_read  dataName='K37_LSD_Relay_EAU1'  dataShape=Scalar  idxSource=Input  idxRow=1  idxCol=1
      settings: SourceProductName=Raptor
  raptor_data_read5 : Raptor_lib/Data Storage/raptor_data_read  dataName='K88_LSD_PWM_Duty'  dataShape=Scalar  idxSource=Input  idxRow=1  idxCol=1
      settings: SourceProductName=Raptor
  raptor_data_read6 : Raptor_lib/Data Storage/raptor_data_read  dataName='K19_LSD_Relay_EAU2'  dataShape=Scalar  idxSource=Input  idxRow=1  idxCol=1
      settings: SourceProductName=Raptor
  raptor_digital_out1 : Raptor_lib/Input & Output/raptor_digital_out  resourceValues=OUTPUT1|OUTPUT2|OUTPUT3|OUTPUT4|OUTPUT5|OUTPUT6|OUTPUT7|OUTPUT8|OUTPUT9|OUTPUT10|OUTPUT11|OUTPUT12|OUTPUT21|OUTPUT22|OUTPUT23|OUTPUT24|OUTPUT25|OUTPUT26|OUTPUT27|OUTPUT28|OUTPUT29|OUTPUT30|OUTPUT31|OUTPUT32|OUTPUT33|OUTPUT34|OUTPUT35|OUTPUT36|OUTPUT37|OUTPUT38|OUTPUT39|OUTPUT40|OUTPUT41|OUTPUT42|OUTPUT43|OUTPUT44|OUTPUT45|OUTPUT46|OUTPUT47|OUTPUT48|OUTPUT49|POWER_HOLD|(None)  resource=OUTPUT34  driverTypeValues=Low Side  driverType=Low Side
      settings: SourceProductName=Raptor
  raptor_digital_out2 : Raptor_lib/Input & Output/raptor_digital_out  resourceValues=OUTPUT1|OUTPUT2|OUTPUT3|OUTPUT4|OUTPUT5|OUTPUT6|OUTPUT7|OUTPUT8|OUTPUT9|OUTPUT10|OUTPUT11|OUTPUT12|OUTPUT21|OUTPUT22|OUTPUT23|OUTPUT24|OUTPUT25|OUTPUT26|OUTPUT27|OUTPUT28|OUTPUT29|OUTPUT30|OUTPUT31|OUTPUT32|OUTPUT33|OUTPUT34|OUTPUT35|OUTPUT36|OUTPUT37|OUTPUT38|OUTPUT39|OUTPUT40|OUTPUT41|OUTPUT42|OUTPUT43|OUTPUT44|OUTPUT45|OUTPUT46|OUTPUT47|OUTPUT48|OUTPUT49|POWER_HOLD|(None)  resource=OUTPUT4  driverTypeValues=Low Side  driverType=Low Side
      settings: SourceProductName=Raptor
  raptor_digital_out3 : Raptor_lib/Input & Output/raptor_digital_out  resourceValues=OUTPUT1|OUTPUT2|OUTPUT3|OUTPUT4|OUTPUT5|OUTPUT6|OUTPUT7|OUTPUT8|OUTPUT9|OUTPUT10|OUTPUT11|OUTPUT12|OUTPUT21|OUTPUT22|OUTPUT23|OUTPUT24|OUTPUT25|OUTPUT26|OUTPUT27|OUTPUT28|OUTPUT29|OUTPUT30|OUTPUT31|OUTPUT32|OUTPUT33|OUTPUT34|OUTPUT35|OUTPUT36|OUTPUT37|OUTPUT38|OUTPUT39|OUTPUT40|OUTPUT41|OUTPUT42|OUTPUT43|OUTPUT44|OUTPUT45|OUTPUT46|OUTPUT47|OUTPUT48|OUTPUT49|POWER_HOLD|(None)  resource=OUTPUT41  driverTypeValues=Low Side  driverType=Low Side
      settings: SourceProductName=Raptor
  raptor_digital_out7 : Raptor_lib/Input & Output/raptor_digital_out  resourceValues=OUTPUT1|OUTPUT2|OUTPUT3|OUTPUT4|OUTPUT5|OUTPUT6|OUTPUT7|OUTPUT8|OUTPUT9|OUTPUT10|OUTPUT11|OUTPUT12|OUTPUT21|OUTPUT22|OUTPUT23|OUTPUT24|OUTPUT25|OUTPUT26|OUTPUT27|OUTPUT28|OUTPUT29|OUTPUT30|OUTPUT31|OUTPUT32|OUTPUT33|OUTPUT34|OUTPUT35|OUTPUT36|OUTPUT37|OUTPUT38|OUTPUT39|OUTPUT40|OUTPUT41|OUTPUT42|OUTPUT43|OUTPUT44|OUTPUT45|OUTPUT46|OUTPUT47|OUTPUT48|OUTPUT49|POWER_HOLD|(None)  resource=OUTPUT23  driverTypeValues=Low Side  driverType=Low Side
      settings: SourceProductName=Raptor
  raptor_override : Raptor_lib/Data Storage/raptor_override  paramName='Cal_Relay_OC'  nameSource=Parameter  measurement=None  calDispType=Number  calEnum={'False', 'True'}  calGain=1.0  calOffset=0.0  calMax=inf  calMin=-inf  calFormat='-1'  calUnit=''  calHelp=''  calAccess=1  calFunction=[raptor_xcp_function(gcb) '|' raptor_get_param_eval(gcb, 'paramName') '_Override']
      settings: SourceProductName=Raptor
  raptor_override1 : Raptor_lib/Data Storage/raptor_override  paramName='Cal_Relay_WC'  nameSource=Parameter  measurement=None  calDispType=Number  calEnum={'False', 'True'}  calGain=1.0  calOffset=0.0  calMax=inf  calMin=-inf  calFormat='-1'  calUnit=''  calHelp=''  calAccess=1  calFunction=[raptor_xcp_function(gcb) '|' raptor_get_param_eval(gcb, 'paramName') '_Override']
      settings: SourceProductName=Raptor
  raptor_override2 : Raptor_lib/Data Storage/raptor_override  paramName='Cal_Relay_EAU1'  nameSource=Parameter  measurement=None  calDispType=Number  calEnum={'False', 'True'}  calGain=1.0  calOffset=0.0  calMax=inf  calMin=-inf  calFormat='-1'  calUnit=''  calHelp=''  calAccess=1  calFunction=[raptor_xcp_function(gcb) '|' raptor_get_param_eval(gcb, 'paramName') '_Override']
      settings: SourceProductName=Raptor
  raptor_override3 : Raptor_lib/Data Storage/raptor_override  paramName='Cal_Relay_EAU2'  nameSource=Parameter  measurement=None  calDispType=Number  calEnum={'False', 'True'}  calGain=1.0  calOffset=0.0  calMax=inf  calMin=-inf  calFormat='-1'  calUnit=''  calHelp=''  calAccess=1  calFunction=[raptor_xcp_function(gcb) '|' raptor_get_param_eval(gcb, 'paramName') '_Override']
      settings: SourceProductName=Raptor
  raptor_pwm_out : Raptor_lib/Input & Output/raptor_pwm_out  showEnable=1  resourceValues=OUTPUT1|OUTPUT2|OUTPUT3|OUTPUT4|OUTPUT5|OUTPUT6|OUTPUT7|OUTPUT8|OUTPUT9|OUTPUT10|OUTPUT11|OUTPUT12|(None)  resource=OUTPUT2  driverTypeValues=Low Side  driverType=Low Side
      settings: SourceProductName=Raptor
  raptor_pwm_out1 : Raptor_lib/Input & Output/raptor_pwm_out  showEnable=1  resourceValues=OUTPUT1|OUTPUT2|OUTPUT3|OUTPUT4|OUTPUT5|OUTPUT6|OUTPUT7|OUTPUT8|OUTPUT9|OUTPUT10|OUTPUT11|OUTPUT12|(None)  resource=OUTPUT6  driverTypeValues=Low Side  driverType=Low Side
      settings: SourceProductName=Raptor
  raptor_pwm_out2 : Raptor_lib/Input & Output/raptor_pwm_out  showEnable=1  resourceValues=OUTPUT1|OUTPUT2|OUTPUT3|OUTPUT4|OUTPUT5|OUTPUT6|OUTPUT7|OUTPUT8|OUTPUT9|OUTPUT10|OUTPUT11|OUTPUT12|(None)  resource=OUTPUT8  driverTypeValues=Low Side  driverType=Low Side
      settings: SourceProductName=Raptor
  wires:
  raptor_adjustment7/1 -> raptor_pwm_out/1
  raptor_adjustment6/1 -> Gain3/1
  raptor_adjustment3/1 -> raptor_pwm_out1/1
  raptor_adjustment8/1 -> Gain5/1
  raptor_data_read/1 -> Gain2/1
  Gain5/1 -> Data Type Conversion3/1
  raptor_data_read1/1 -> Gain4/1
  Gain3/1 -> Data Type Conversion1/1
  Data Type Conversion1/1 -> raptor_pwm_out/3
  Data Type Conversion3/1 -> raptor_pwm_out1/3
  Data Type Conversion/1 -> raptor_pwm_out/2
  Data Type Conversion2/1 -> raptor_pwm_out1/2
  Gain2/1 -> Data Type Conversion2/1
  Gain4/1 -> Data Type Conversion/1
  raptor_data_read2/1 -> raptor_override/1
  raptor_data_read6/1 -> raptor_override3/1
  raptor_data_read3/1 -> raptor_override1/1
  raptor_data_read4/1 -> raptor_override2/1
  Gain6/1 -> Data Type Conversion4/1
  Data Type Conversion4/1 -> raptor_pwm_out2/2
  Data Type Conversion5/1 -> raptor_pwm_out2/3
  Gain1/1 -> Data Type Conversion5/1
  raptor_data_read5/1 -> Gain6/1
  raptor_adjustment1/1 -> Gain1/1
  raptor_adjustment2/1 -> raptor_pwm_out2/1
  raptor_override/1 -> raptor_digital_out2/1
  raptor_override1/1 -> raptor_digital_out3/1
  raptor_override2/1 -> raptor_digital_out7/1
  raptor_override3/1 -> raptor_digital_out1/1

== system EPT/I//O/Output/Curtis_Reserved  ==
  raptor_adjustment1 : Raptor_lib/Data Storage/raptor_adjustment  paramName='K53_HSD_Reverse'  nameSource=Parameter  initValue=0.00  dataType=boolean  storage=Calibration  calDispType=Number  calEnum={'False', 'True'}  calGain=1.0  calOffset=0.0  calMax=inf  calMin=-inf  calFormat='-1'  calUnit=''  calHelp=''  calAccess=1  calFunction=raptor_xcp_function(gcb)  calDispHeaders=off  calColHeaders={'Col1' 'Col2' 'Col3'}  calRowHeaders={'Row1' 'Row2' 'Row3'}
      settings: SourceProductName=Raptor
  raptor_adjustment3 : Raptor_lib/Data Storage/raptor_adjustment  paramName='K89_HSD_Forward'  nameSource=Parameter  initValue=0.00  dataType=boolean  storage=Calibration  calDispType=Number  calEnum={'False', 'True'}  calGain=1.0  calOffset=0.0  calMax=inf  calMin=-inf  calFormat='-1'  calUnit=''  calHelp=''  calAccess=1  calFunction=raptor_xcp_function(gcb)  calDispHeaders=off  calColHeaders={'Col1' 'Col2' 'Col3'}  calRowHeaders={'Row1' 'Row2' 'Row3'}
      settings: SourceProductName=Raptor
  raptor_digital_out1 : Raptor_lib/Input & Output/raptor_digital_out  resourceValues=OUTPUT1|OUTPUT2|OUTPUT3|OUTPUT4|OUTPUT5|OUTPUT6|OUTPUT7|OUTPUT8|OUTPUT9|OUTPUT10|OUTPUT11|OUTPUT12|OUTPUT21|OUTPUT22|OUTPUT23|OUTPUT24|OUTPUT25|OUTPUT26|OUTPUT27|OUTPUT28|OUTPUT29|OUTPUT30|OUTPUT31|OUTPUT32|OUTPUT33|OUTPUT34|OUTPUT35|OUTPUT36|OUTPUT37|OUTPUT38|OUTPUT39|OUTPUT40|OUTPUT41|OUTPUT42|OUTPUT43|OUTPUT44|OUTPUT45|OUTPUT46|OUTPUT47|OUTPUT48|OUTPUT49|POWER_HOLD|(None)  resource=OUTPUT49  driverTypeValues=High Side  driverType=High Side
      settings: SourceProductName=Raptor
  raptor_digital_out3 : Raptor_lib/Input & Output/raptor_digital_out  resourceValues=OUTPUT1|OUTPUT2|OUTPUT3|OUTPUT4|OUTPUT5|OUTPUT6|OUTPUT7|OUTPUT8|OUTPUT9|OUTPUT10|OUTPUT11|OUTPUT12|OUTPUT21|OUTPUT22|OUTPUT23|OUTPUT24|OUTPUT25|OUTPUT26|OUTPUT27|OUTPUT28|OUTPUT29|OUTPUT30|OUTPUT31|OUTPUT32|OUTPUT33|OUTPUT34|OUTPUT35|OUTPUT36|OUTPUT37|OUTPUT38|OUTPUT39|OUTPUT40|OUTPUT41|OUTPUT42|OUTPUT43|OUTPUT44|OUTPUT45|OUTPUT46|OUTPUT47|OUTPUT48|OUTPUT49|POWER_HOLD|(None)  resource=OUTPUT48  driverTypeValues=High Side  driverType=High Side
      settings: SourceProductName=Raptor
  wires:
  raptor_adjustment3/1 -> raptor_digital_out3/1
  raptor_adjustment1/1 -> raptor_digital_out1/1
